simulink model "TST_DrvDem_CalcState"  (R2016b)
settings: Solver=FixedStepDiscrete  StartTime=0.0  StopTime=simTime  FixedStep=sampleTime  RelTol=1e-3
values from neighbouring files (symbols this model uses):
  testCase = 1    [initTST_DrvDem_CalcState_001.m]    (also in initTST_DrvDem_CalcState_002.m = 2)
libraries: simulink x11, UnitTest_Lib x8
settings Model: Creator=zhengjinyan  LastModifiedBy=zhengjinyan
settings DebuggingCC: SignalRangeChecking=error

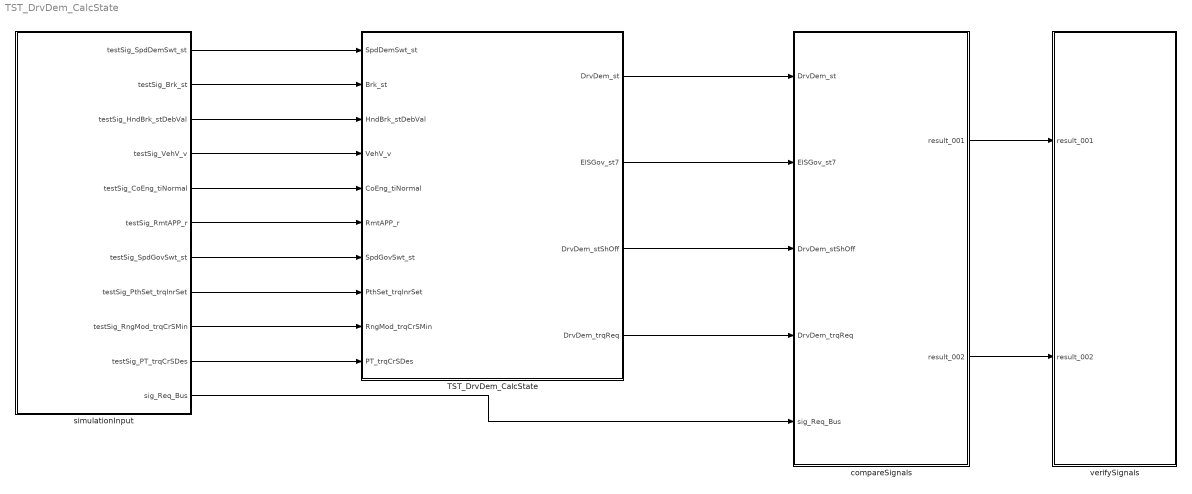
== system TST_DrvDem_CalcState ==
  TST_DrvDem_CalcState : Subsystem
  compareSignals : Subsystem
  simulationInput : Subsystem
  verifySignals : Subsystem
  wires:
  simulationInput/1(testSig_SpdDemSwt_st) -> TST_DrvDem_CalcState/1(SpdDemSwt_st)
  simulationInput/2(testSig_Brk_st) -> TST_DrvDem_CalcState/2(Brk_st)
  simulationInput/3(testSig_HndBrk_stDebVal) -> TST_DrvDem_CalcState/3(HndBrk_stDebVal)
  simulationInput/4(testSig_VehV_v) -> TST_DrvDem_CalcState/4(VehV_v)
  simulationInput/5(testSig_CoEng_tiNormal) -> TST_DrvDem_CalcState/5(CoEng_tiNormal)
  simulationInput/6(testSig_RmtAPP_r) -> TST_DrvDem_CalcState/6(RmtAPP_r)
  simulationInput/7(testSig_SpdGovSwt_st) -> TST_DrvDem_CalcState/7(SpdGovSwt_st)
  simulationInput/8(testSig_PthSet_trqInrSet) -> TST_DrvDem_CalcState/8(PthSet_trqInrSet)
  simulationInput/9(testSig_RngMod_trqCrSMin) -> TST_DrvDem_CalcState/9(RngMod_trqCrSMin)
  simulationInput/10(testSig_PT_trqCrSDes) -> TST_DrvDem_CalcState/10(PT_trqCrSDes)
  TST_DrvDem_CalcState/1(DrvDem_st) -> compareSignals/1(DrvDem_st)
  TST_DrvDem_CalcState/2(EISGov_st7) -> compareSignals/2(EISGov_st7)
  TST_DrvDem_CalcState/3(DrvDem_stShOff) -> compareSignals/3(DrvDem_stShOff)
  TST_DrvDem_CalcState/4(DrvDem_trqReq) -> compareSignals/4(DrvDem_trqReq)
  simulationInput/11(sig_Req_Bus) -> compareSignals/5(sig_Req_Bus)
  compareSignals/1(result_001) -> verifySignals/1(result_001)
  compareSignals/2(result_002) -> verifySignals/2(result_002)

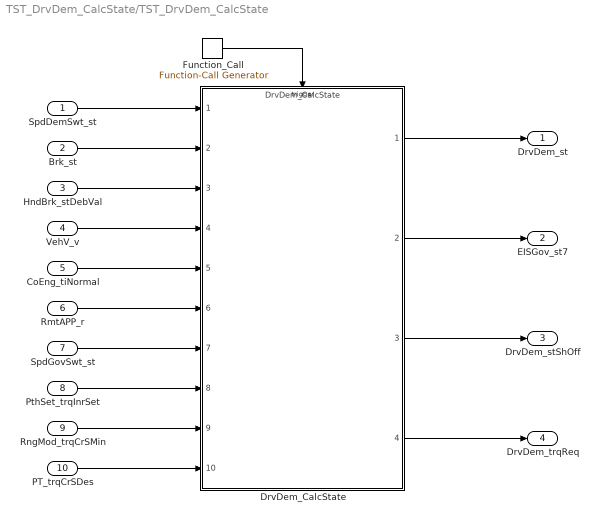
== system TST_DrvDem_CalcState/TST_DrvDem_CalcState ==
  SpdDemSwt_st : Inport
  Brk_st : Inport  Port=2
  HndBrk_stDebVal : Inport  Port=3
  VehV_v : Inport  Port=4
  CoEng_tiNormal : Inport  Port=5
  RmtAPP_r : Inport  Port=6
  SpdGovSwt_st : Inport  Port=7
  PthSet_trqInrSet : Inport  Port=8
  RngMod_trqCrSMin : Inport  Port=9
  PT_trqCrSDes : Inport  Port=10
  DrvDem_CalcState : ModelReference  ModelNameDialog=DrvDem_CalcState  SimulationMode=Normal  ModelReferenceVersion=1.66  TriggerPortName=function  TriggerPortTriggerType=function-call  TriggerPortStatesWhenEnabling=held
  Function_Call : simulink/Ports & Subsystems/Function-Call Generator  sample_time=sampleTime  numberOfIterations=1
  DrvDem_st : Outport
  EISGov_st7 : Outport  Port=2
  DrvDem_stShOff : Outport  Port=3
  DrvDem_trqReq : Outport  Port=4
  wires:
  Function_Call/1 -> DrvDem_CalcState/Trigger
  SpdDemSwt_st/1 -> DrvDem_CalcState/1
  Brk_st/1 -> DrvDem_CalcState/2
  HndBrk_stDebVal/1 -> DrvDem_CalcState/3
  VehV_v/1 -> DrvDem_CalcState/4
  CoEng_tiNormal/1 -> DrvDem_CalcState/5
  RmtAPP_r/1 -> DrvDem_CalcState/6
  SpdGovSwt_st/1 -> DrvDem_CalcState/7
  PthSet_trqInrSet/1 -> DrvDem_CalcState/8
  RngMod_trqCrSMin/1 -> DrvDem_CalcState/9
  PT_trqCrSDes/1 -> DrvDem_CalcState/10
  DrvDem_CalcState/1 -> DrvDem_st/1
  DrvDem_CalcState/2 -> EISGov_st7/1
  DrvDem_CalcState/3 -> DrvDem_stShOff/1
  DrvDem_CalcState/4 -> DrvDem_trqReq/1

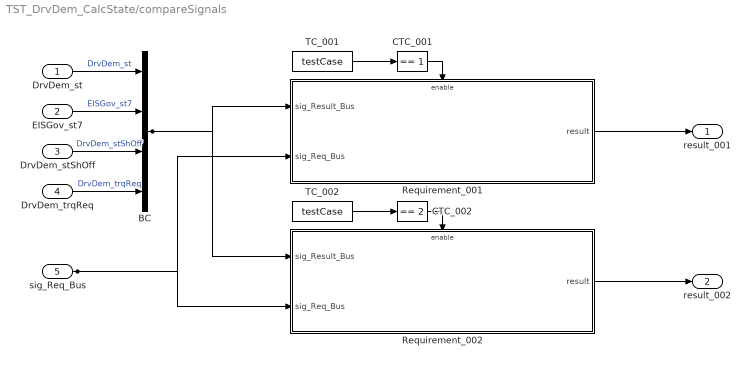
== system TST_DrvDem_CalcState/compareSignals ==
  DrvDem_st : Inport
  EISGov_st7 : Inport  Port=2
  DrvDem_stShOff : Inport  Port=3
  DrvDem_trqReq : Inport  Port=4
  sig_Req_Bus : Inport  Port=5
  BC : BusCreator  Inputs=4
  CTC_001 : simulink/Logic and Bit Operations/Compare To Constant  relop===  const=1  OutDataTypeStr=boolean
  CTC_002 : simulink/Logic and Bit Operations/Compare To Constant  relop===  const=2  OutDataTypeStr=boolean
  Requirement_001 : Subsystem
  Requirement_002 : Subsystem
  TC_001 : Constant  Value=testCase
  TC_002 : Constant  Value=testCase
  result_001 : Outport
  result_002 : Outport  Port=2
  wires:
  DrvDem_st/1 -> BC/1  "DrvDem_st"
  EISGov_st7/1 -> BC/2  "EISGov_st7"
  DrvDem_stShOff/1 -> BC/3  "DrvDem_stShOff"
  DrvDem_trqReq/1 -> BC/4  "DrvDem_trqReq"
  TC_001/1 -> CTC_001/1
  CTC_001/1 -> Requirement_001/Enable
  sig_Req_Bus/1 -> Requirement_001/2(sig_Req_Bus), Requirement_002/2(sig_Req_Bus)
  BC/1 -> Requirement_001/1(sig_Result_Bus), Requirement_002/1(sig_Result_Bus)
  Requirement_001/1(result) -> result_001/1
  TC_002/1 -> CTC_002/1
  CTC_002/1 -> Requirement_002/Enable
  Requirement_002/1(result) -> result_002/1

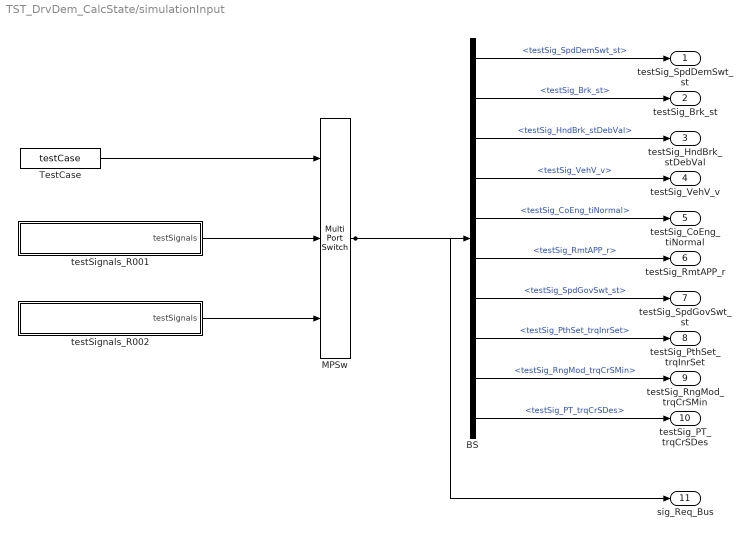
== system TST_DrvDem_CalcState/simulationInput ==
  BS : BusSelector  OutputSignals=testSig_SpdDemSwt_st,testSig_Brk_st,testSig_HndBrk_stDebVal,testSig_VehV_v,testSig_CoEng_tiNormal,testSig_RmtAPP_r,testSig_SpdGovSwt_st,testSig_PthSet_trqInrSet,testSig_RngMod_trqCrSMin,testSig_PT_trqCrSDes
  MPSw : MultiPortSwitch  Inputs=2  SaturateOnIntegerOverflow=on  InputSameDT=on
  TestCase : Constant  Value=testCase
  testSignals_R001 : Subsystem
  testSignals_R002 : Subsystem
  testSig_SpdDemSwt_st : Outport
  testSig_Brk_st : Outport  Port=2
  testSig_HndBrk_stDebVal : Outport  Port=3
  testSig_VehV_v : Outport  Port=4
  testSig_CoEng_tiNormal : Outport  Port=5
  testSig_RmtAPP_r : Outport  Port=6
  testSig_SpdGovSwt_st : Outport  Port=7
  testSig_PthSet_trqInrSet : Outport  Port=8
  testSig_RngMod_trqCrSMin : Outport  Port=9
  testSig_PT_trqCrSDes : Outport  Port=10
  sig_Req_Bus : Outport  Port=11
  wires:
  BS/1 -> testSig_SpdDemSwt_st/1  "<testSig_SpdDemSwt_st>"
  BS/2 -> testSig_Brk_st/1  "<testSig_Brk_st>"
  BS/3 -> testSig_HndBrk_stDebVal/1  "<testSig_HndBrk_stDebVal>"
  BS/4 -> testSig_VehV_v/1  "<testSig_VehV_v>"
  BS/5 -> testSig_CoEng_tiNormal/1  "<testSig_CoEng_tiNormal>"
  BS/6 -> testSig_RmtAPP_r/1  "<testSig_RmtAPP_r>"
  BS/7 -> testSig_SpdGovSwt_st/1  "<testSig_SpdGovSwt_st>"
  BS/8 -> testSig_PthSet_trqInrSet/1  "<testSig_PthSet_trqInrSet>"
  BS/9 -> testSig_RngMod_trqCrSMin/1  "<testSig_RngMod_trqCrSMin>"
  BS/10 -> testSig_PT_trqCrSDes/1  "<testSig_PT_trqCrSDes>"
  MPSw/1 -> BS/1, sig_Req_Bus/1
  TestCase/1 -> MPSw/1
  testSignals_R001/1(testSignals) -> MPSw/2
  testSignals_R002/1(testSignals) -> MPSw/3

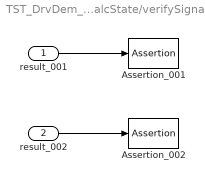
== system TST_DrvDem_CalcState/verifySignals ==
  result_001 : Inport
  result_002 : Inport  Port=2
  Assertion_001 : Assertion  Enabled=off
  Assertion_002 : Assertion  Enabled=off
  wires:
  result_001/1 -> Assertion_001/1
  result_002/1 -> Assertion_002/1

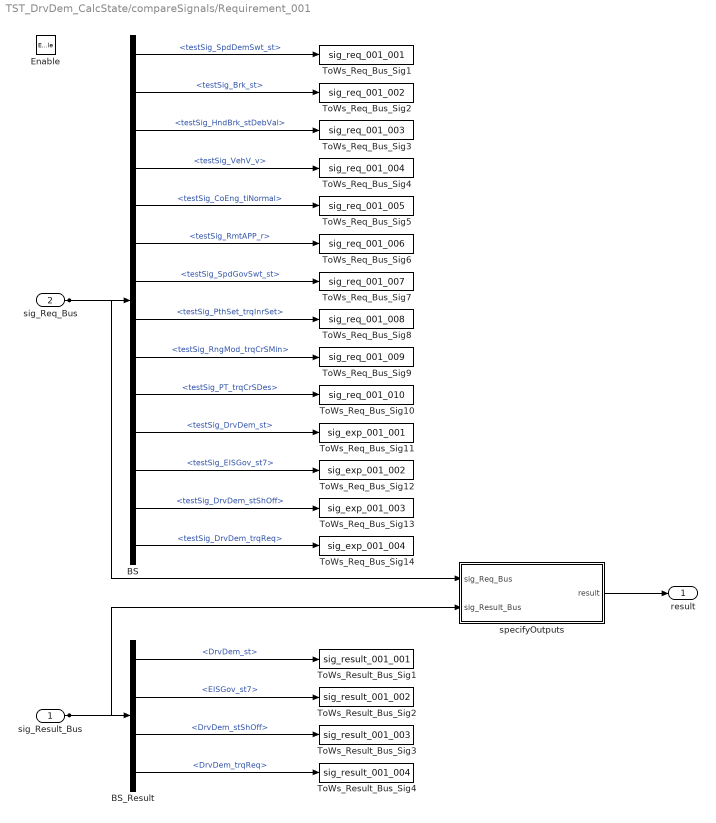
== system TST_DrvDem_CalcState/compareSignals/Requirement_001 ==
  sig_Result_Bus : Inport
  sig_Req_Bus : Inport  Port=2
  Enable : EnablePort
  BS : BusSelector  OutputSignals=testSig_SpdDemSwt_st,testSig_Brk_st,testSig_HndBrk_stDebVal,testSig_VehV_v,testSig_CoEng_tiNormal,testSig_RmtAPP_r,testSig_SpdGovSwt_st,testSig_PthSet_trqInrSet,testSig_RngMod_trqCrSMin,testSig_PT_trqCrSDes,testSig_DrvDem_st,testSig_EISGov_st7,testSig_DrvDem_stShOff,testSig_DrvDem_trqReq
  BS_Result : BusSelector  OutputSignals=DrvDem_st,EISGov_st7,DrvDem_stShOff,DrvDem_trqReq
  ToWs_Req_Bus_Sig1 : ToWorkspace  VariableName=sig_req_001_001  SaveFormat=Structure With Time
  ToWs_Req_Bus_Sig10 : ToWorkspace  VariableName=sig_req_001_010  SaveFormat=Structure With Time
  ToWs_Req_Bus_Sig11 : ToWorkspace  VariableName=sig_exp_001_001  SaveFormat=Structure With Time
  ToWs_Req_Bus_Sig12 : ToWorkspace  VariableName=sig_exp_001_002  SaveFormat=Structure With Time
  ToWs_Req_Bus_Sig13 : ToWorkspace  VariableName=sig_exp_001_003  SaveFormat=Structure With Time
  ToWs_Req_Bus_Sig14 : ToWorkspace  VariableName=sig_exp_001_004  SaveFormat=Structure With Time
  ToWs_Req_Bus_Sig2 : ToWorkspace  VariableName=sig_req_001_002  SaveFormat=Structure With Time
  ToWs_Req_Bus_Sig3 : ToWorkspace  VariableName=sig_req_001_003  SaveFormat=Structure With Time
  ToWs_Req_Bus_Sig4 : ToWorkspace  VariableName=sig_req_001_004  SaveFormat=Structure With Time
  ToWs_Req_Bus_Sig5 : ToWorkspace  VariableName=sig_req_001_005  SaveFormat=Structure With Time
  ToWs_Req_Bus_Sig6 : ToWorkspace  VariableName=sig_req_001_006  SaveFormat=Structure With Time
  ToWs_Req_Bus_Sig7 : ToWorkspace  VariableName=sig_req_001_007  SaveFormat=Structure With Time
  ToWs_Req_Bus_Sig8 : ToWorkspace  VariableName=sig_req_001_008  SaveFormat=Structure With Time
  ToWs_Req_Bus_Sig9 : ToWorkspace  VariableName=sig_req_001_009  SaveFormat=Structure With Time
  ToWs_Result_Bus_Sig1 : ToWorkspace  VariableName=sig_result_001_001  SaveFormat=Structure With Time
  ToWs_Result_Bus_Sig2 : ToWorkspace  VariableName=sig_result_001_002  SaveFormat=Structure With Time
  ToWs_Result_Bus_Sig3 : ToWorkspace  VariableName=sig_result_001_003  SaveFormat=Structure With Time
  ToWs_Result_Bus_Sig4 : ToWorkspace  VariableName=sig_result_001_004  SaveFormat=Structure With Time
  specifyOutputs : Subsystem
  result : Outport
  wires:
  sig_Req_Bus/1 -> BS/1, specifyOutputs/1(sig_Req_Bus)
  BS/1 -> ToWs_Req_Bus_Sig1/1  "<testSig_SpdDemSwt_st>"
  BS/2 -> ToWs_Req_Bus_Sig2/1  "<testSig_Brk_st>"
  BS/3 -> ToWs_Req_Bus_Sig3/1  "<testSig_HndBrk_stDebVal>"
  BS/4 -> ToWs_Req_Bus_Sig4/1  "<testSig_VehV_v>"
  BS/5 -> ToWs_Req_Bus_Sig5/1  "<testSig_CoEng_tiNormal>"
  BS/6 -> ToWs_Req_Bus_Sig6/1  "<testSig_RmtAPP_r>"
  BS/7 -> ToWs_Req_Bus_Sig7/1  "<testSig_SpdGovSwt_st>"
  BS/8 -> ToWs_Req_Bus_Sig8/1  "<testSig_PthSet_trqInrSet>"
  BS/9 -> ToWs_Req_Bus_Sig9/1  "<testSig_RngMod_trqCrSMin>"
  BS/10 -> ToWs_Req_Bus_Sig10/1  "<testSig_PT_trqCrSDes>"
  BS/11 -> ToWs_Req_Bus_Sig11/1  "<testSig_DrvDem_st>"
  BS/12 -> ToWs_Req_Bus_Sig12/1  "<testSig_EISGov_st7>"
  BS/13 -> ToWs_Req_Bus_Sig13/1  "<testSig_DrvDem_stShOff>"
  BS/14 -> ToWs_Req_Bus_Sig14/1  "<testSig_DrvDem_trqReq>"
  sig_Result_Bus/1 -> BS_Result/1, specifyOutputs/2(sig_Result_Bus)
  BS_Result/1 -> ToWs_Result_Bus_Sig1/1  "<DrvDem_st>"
  BS_Result/2 -> ToWs_Result_Bus_Sig2/1  "<EISGov_st7>"
  BS_Result/3 -> ToWs_Result_Bus_Sig3/1  "<DrvDem_stShOff>"
  BS_Result/4 -> ToWs_Result_Bus_Sig4/1  "<DrvDem_trqReq>"
  specifyOutputs/1(result) -> result/1

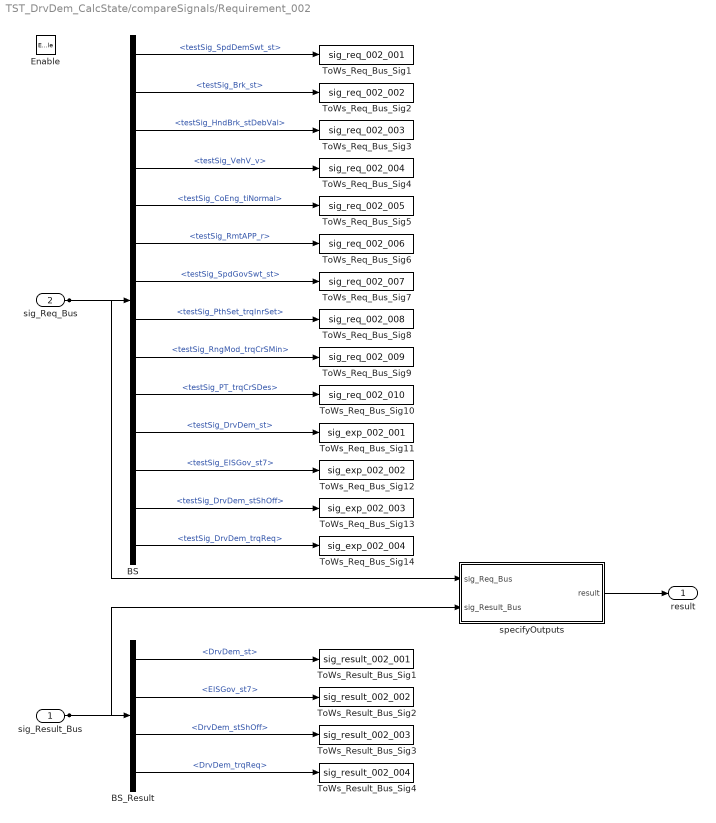
== system TST_DrvDem_CalcState/compareSignals/Requirement_002 ==
  sig_Result_Bus : Inport
  sig_Req_Bus : Inport  Port=2
  Enable : EnablePort
  BS : BusSelector  OutputSignals=testSig_SpdDemSwt_st,testSig_Brk_st,testSig_HndBrk_stDebVal,testSig_VehV_v,testSig_CoEng_tiNormal,testSig_RmtAPP_r,testSig_SpdGovSwt_st,testSig_PthSet_trqInrSet,testSig_RngMod_trqCrSMin,testSig_PT_trqCrSDes,testSig_DrvDem_st,testSig_EISGov_st7,testSig_DrvDem_stShOff,testSig_DrvDem_trqReq
  BS_Result : BusSelector  OutputSignals=DrvDem_st,EISGov_st7,DrvDem_stShOff,DrvDem_trqReq
  ToWs_Req_Bus_Sig1 : ToWorkspace  VariableName=sig_req_002_001  SaveFormat=Structure With Time
  ToWs_Req_Bus_Sig10 : ToWorkspace  VariableName=sig_req_002_010  SaveFormat=Structure With Time
  ToWs_Req_Bus_Sig11 : ToWorkspace  VariableName=sig_exp_002_001  SaveFormat=Structure With Time
  ToWs_Req_Bus_Sig12 : ToWorkspace  VariableName=sig_exp_002_002  SaveFormat=Structure With Time
  ToWs_Req_Bus_Sig13 : ToWorkspace  VariableName=sig_exp_002_003  SaveFormat=Structure With Time
  ToWs_Req_Bus_Sig14 : ToWorkspace  VariableName=sig_exp_002_004  SaveFormat=Structure With Time
  ToWs_Req_Bus_Sig2 : ToWorkspace  VariableName=sig_req_002_002  SaveFormat=Structure With Time
  ToWs_Req_Bus_Sig3 : ToWorkspace  VariableName=sig_req_002_003  SaveFormat=Structure With Time
  ToWs_Req_Bus_Sig4 : ToWorkspace  VariableName=sig_req_002_004  SaveFormat=Structure With Time
  ToWs_Req_Bus_Sig5 : ToWorkspace  VariableName=sig_req_002_005  SaveFormat=Structure With Time
  ToWs_Req_Bus_Sig6 : ToWorkspace  VariableName=sig_req_002_006  SaveFormat=Structure With Time
  ToWs_Req_Bus_Sig7 : ToWorkspace  VariableName=sig_req_002_007  SaveFormat=Structure With Time
  ToWs_Req_Bus_Sig8 : ToWorkspace  VariableName=sig_req_002_008  SaveFormat=Structure With Time
  ToWs_Req_Bus_Sig9 : ToWorkspace  VariableName=sig_req_002_009  SaveFormat=Structure With Time
  ToWs_Result_Bus_Sig1 : ToWorkspace  VariableName=sig_result_002_001  SaveFormat=Structure With Time
  ToWs_Result_Bus_Sig2 : ToWorkspace  VariableName=sig_result_002_002  SaveFormat=Structure With Time
  ToWs_Result_Bus_Sig3 : ToWorkspace  VariableName=sig_result_002_003  SaveFormat=Structure With Time
  ToWs_Result_Bus_Sig4 : ToWorkspace  VariableName=sig_result_002_004  SaveFormat=Structure With Time
  specifyOutputs : Subsystem
  result : Outport
  wires:
  sig_Req_Bus/1 -> BS/1, specifyOutputs/1(sig_Req_Bus)
  BS/1 -> ToWs_Req_Bus_Sig1/1  "<testSig_SpdDemSwt_st>"
  BS/2 -> ToWs_Req_Bus_Sig2/1  "<testSig_Brk_st>"
  BS/3 -> ToWs_Req_Bus_Sig3/1  "<testSig_HndBrk_stDebVal>"
  BS/4 -> ToWs_Req_Bus_Sig4/1  "<testSig_VehV_v>"
  BS/5 -> ToWs_Req_Bus_Sig5/1  "<testSig_CoEng_tiNormal>"
  BS/6 -> ToWs_Req_Bus_Sig6/1  "<testSig_RmtAPP_r>"
  BS/7 -> ToWs_Req_Bus_Sig7/1  "<testSig_SpdGovSwt_st>"
  BS/8 -> ToWs_Req_Bus_Sig8/1  "<testSig_PthSet_trqInrSet>"
  BS/9 -> ToWs_Req_Bus_Sig9/1  "<testSig_RngMod_trqCrSMin>"
  BS/10 -> ToWs_Req_Bus_Sig10/1  "<testSig_PT_trqCrSDes>"
  BS/11 -> ToWs_Req_Bus_Sig11/1  "<testSig_DrvDem_st>"
  BS/12 -> ToWs_Req_Bus_Sig12/1  "<testSig_EISGov_st7>"
  BS/13 -> ToWs_Req_Bus_Sig13/1  "<testSig_DrvDem_stShOff>"
  BS/14 -> ToWs_Req_Bus_Sig14/1  "<testSig_DrvDem_trqReq>"
  sig_Result_Bus/1 -> BS_Result/1, specifyOutputs/2(sig_Result_Bus)
  BS_Result/1 -> ToWs_Result_Bus_Sig1/1  "<DrvDem_st>"
  BS_Result/2 -> ToWs_Result_Bus_Sig2/1  "<EISGov_st7>"
  BS_Result/3 -> ToWs_Result_Bus_Sig3/1  "<DrvDem_stShOff>"
  BS_Result/4 -> ToWs_Result_Bus_Sig4/1  "<DrvDem_trqReq>"
  specifyOutputs/1(result) -> result/1

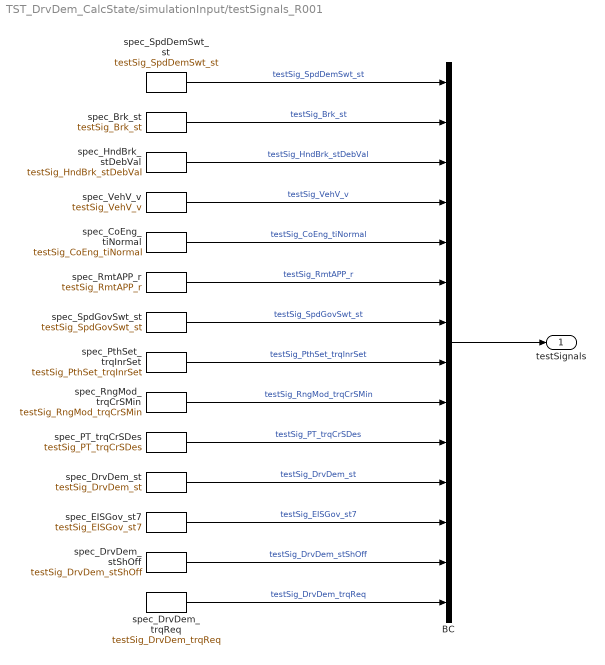
== system TST_DrvDem_CalcState/simulationInput/testSignals_R001 ==
  BC : BusCreator  Inputs=14
  spec_Brk_st : FromWorkspace  VariableName=testSig_Brk_st  Interpolate=off  OutputAfterFinalValue=Holding final value
  spec_CoEng_tiNormal : FromWorkspace  VariableName=testSig_CoEng_tiNormal  Interpolate=off  OutputAfterFinalValue=Holding final value
  spec_DrvDem_st : FromWorkspace  VariableName=testSig_DrvDem_st  Interpolate=off  OutputAfterFinalValue=Holding final value
  spec_DrvDem_stShOff : FromWorkspace  VariableName=testSig_DrvDem_stShOff  Interpolate=off  OutputAfterFinalValue=Holding final value
  spec_DrvDem_trqReq : FromWorkspace  VariableName=testSig_DrvDem_trqReq  Interpolate=off  OutputAfterFinalValue=Holding final value
  spec_EISGov_st7 : FromWorkspace  VariableName=testSig_EISGov_st7  Interpolate=off  OutputAfterFinalValue=Holding final value
  spec_HndBrk_stDebVal : FromWorkspace  VariableName=testSig_HndBrk_stDebVal  Interpolate=off  OutputAfterFinalValue=Holding final value
  spec_PT_trqCrSDes : FromWorkspace  VariableName=testSig_PT_trqCrSDes  Interpolate=off  OutputAfterFinalValue=Holding final value
  spec_PthSet_trqInrSet : FromWorkspace  VariableName=testSig_PthSet_trqInrSet  Interpolate=off  OutputAfterFinalValue=Holding final value
  spec_RmtAPP_r : FromWorkspace  VariableName=testSig_RmtAPP_r  Interpolate=off  OutputAfterFinalValue=Holding final value
  spec_RngMod_trqCrSMin : FromWorkspace  VariableName=testSig_RngMod_trqCrSMin  Interpolate=off  OutputAfterFinalValue=Holding final value
  spec_SpdDemSwt_st : FromWorkspace  VariableName=testSig_SpdDemSwt_st  Interpolate=off  OutputAfterFinalValue=Holding final value
  spec_SpdGovSwt_st : FromWorkspace  VariableName=testSig_SpdGovSwt_st  Interpolate=off  OutputAfterFinalValue=Holding final value
  spec_VehV_v : FromWorkspace  VariableName=testSig_VehV_v  Interpolate=off  OutputAfterFinalValue=Holding final value
  testSignals : Outport
  wires:
  BC/1 -> testSignals/1
  spec_SpdDemSwt_st/1 -> BC/1  "testSig_SpdDemSwt_st"
  spec_Brk_st/1 -> BC/2  "testSig_Brk_st"
  spec_HndBrk_stDebVal/1 -> BC/3  "testSig_HndBrk_stDebVal"
  spec_VehV_v/1 -> BC/4  "testSig_VehV_v"
  spec_CoEng_tiNormal/1 -> BC/5  "testSig_CoEng_tiNormal"
  spec_RmtAPP_r/1 -> BC/6  "testSig_RmtAPP_r"
  spec_SpdGovSwt_st/1 -> BC/7  "testSig_SpdGovSwt_st"
  spec_PthSet_trqInrSet/1 -> BC/8  "testSig_PthSet_trqInrSet"
  spec_RngMod_trqCrSMin/1 -> BC/9  "testSig_RngMod_trqCrSMin"
  spec_PT_trqCrSDes/1 -> BC/10  "testSig_PT_trqCrSDes"
  spec_DrvDem_st/1 -> BC/11  "testSig_DrvDem_st"
  spec_EISGov_st7/1 -> BC/12  "testSig_EISGov_st7"
  spec_DrvDem_stShOff/1 -> BC/13  "testSig_DrvDem_stShOff"
  spec_DrvDem_trqReq/1 -> BC/14  "testSig_DrvDem_trqReq"

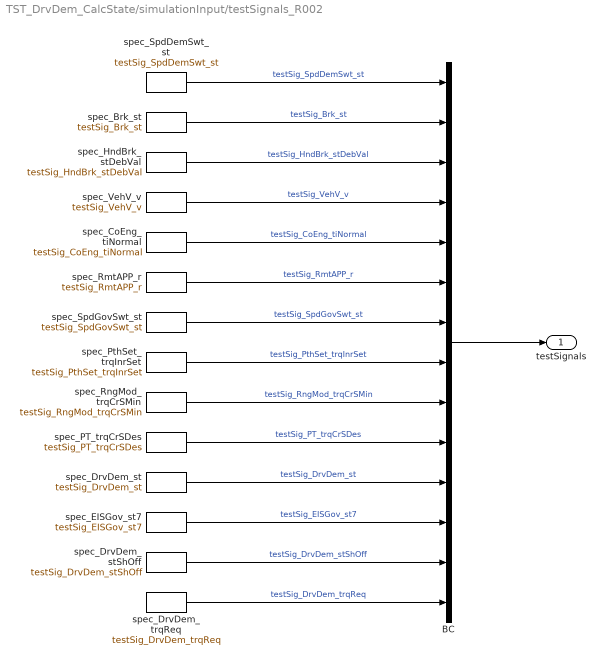
== system TST_DrvDem_CalcState/simulationInput/testSignals_R002 ==
  BC : BusCreator  Inputs=14
  spec_Brk_st : FromWorkspace  VariableName=testSig_Brk_st  Interpolate=off  OutputAfterFinalValue=Holding final value
  spec_CoEng_tiNormal : FromWorkspace  VariableName=testSig_CoEng_tiNormal  Interpolate=off  OutputAfterFinalValue=Holding final value
  spec_DrvDem_st : FromWorkspace  VariableName=testSig_DrvDem_st  Interpolate=off  OutputAfterFinalValue=Holding final value
  spec_DrvDem_stShOff : FromWorkspace  VariableName=testSig_DrvDem_stShOff  Interpolate=off  OutputAfterFinalValue=Holding final value
  spec_DrvDem_trqReq : FromWorkspace  VariableName=testSig_DrvDem_trqReq  Interpolate=off  OutputAfterFinalValue=Holding final value
  spec_EISGov_st7 : FromWorkspace  VariableName=testSig_EISGov_st7  Interpolate=off  OutputAfterFinalValue=Holding final value
  spec_HndBrk_stDebVal : FromWorkspace  VariableName=testSig_HndBrk_stDebVal  Interpolate=off  OutputAfterFinalValue=Holding final value
  spec_PT_trqCrSDes : FromWorkspace  VariableName=testSig_PT_trqCrSDes  Interpolate=off  OutputAfterFinalValue=Holding final value
  spec_PthSet_trqInrSet : FromWorkspace  VariableName=testSig_PthSet_trqInrSet  Interpolate=off  OutputAfterFinalValue=Holding final value
  spec_RmtAPP_r : FromWorkspace  VariableName=testSig_RmtAPP_r  Interpolate=off  OutputAfterFinalValue=Holding final value
  spec_RngMod_trqCrSMin : FromWorkspace  VariableName=testSig_RngMod_trqCrSMin  Interpolate=off  OutputAfterFinalValue=Holding final value
  spec_SpdDemSwt_st : FromWorkspace  VariableName=testSig_SpdDemSwt_st  Interpolate=off  OutputAfterFinalValue=Holding final value
  spec_SpdGovSwt_st : FromWorkspace  VariableName=testSig_SpdGovSwt_st  Interpolate=off  OutputAfterFinalValue=Holding final value
  spec_VehV_v : FromWorkspace  VariableName=testSig_VehV_v  Interpolate=off  OutputAfterFinalValue=Holding final value
  testSignals : Outport
  wires:
  BC/1 -> testSignals/1
  spec_SpdDemSwt_st/1 -> BC/1  "testSig_SpdDemSwt_st"
  spec_Brk_st/1 -> BC/2  "testSig_Brk_st"
  spec_HndBrk_stDebVal/1 -> BC/3  "testSig_HndBrk_stDebVal"
  spec_VehV_v/1 -> BC/4  "testSig_VehV_v"
  spec_CoEng_tiNormal/1 -> BC/5  "testSig_CoEng_tiNormal"
  spec_RmtAPP_r/1 -> BC/6  "testSig_RmtAPP_r"
  spec_SpdGovSwt_st/1 -> BC/7  "testSig_SpdGovSwt_st"
  spec_PthSet_trqInrSet/1 -> BC/8  "testSig_PthSet_trqInrSet"
  spec_RngMod_trqCrSMin/1 -> BC/9  "testSig_RngMod_trqCrSMin"
  spec_PT_trqCrSDes/1 -> BC/10  "testSig_PT_trqCrSDes"
  spec_DrvDem_st/1 -> BC/11  "testSig_DrvDem_st"
  spec_EISGov_st7/1 -> BC/12  "testSig_EISGov_st7"
  spec_DrvDem_stShOff/1 -> BC/13  "testSig_DrvDem_stShOff"
  spec_DrvDem_trqReq/1 -> BC/14  "testSig_DrvDem_trqReq"

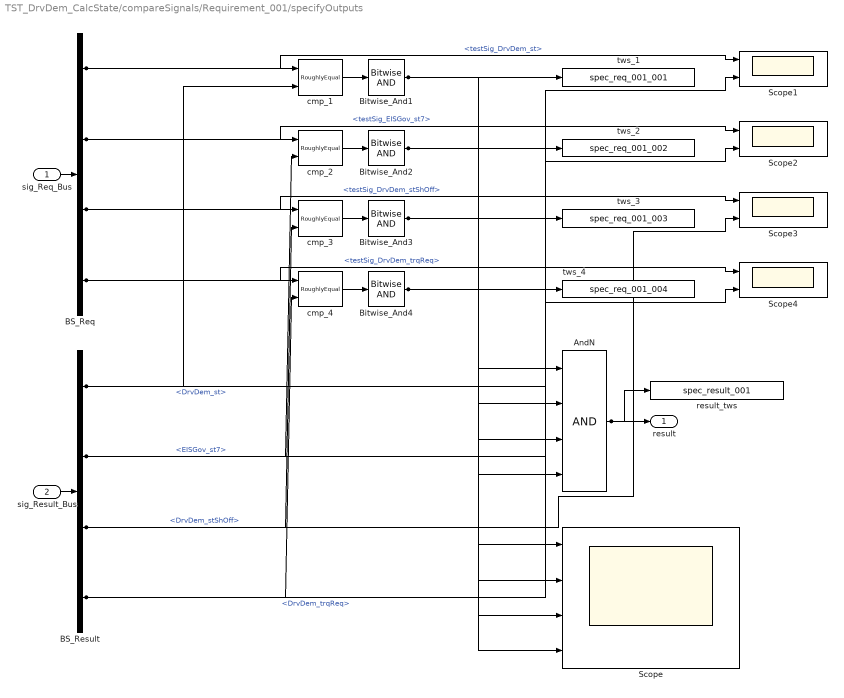
== system TST_DrvDem_CalcState/compareSignals/Requirement_001/specifyOutputs ==
  sig_Req_Bus : Inport
  sig_Result_Bus : Inport  Port=2
  AndN : Logic  Inputs=4
  BS_Req : BusSelector  OutputSignals=testSig_DrvDem_st,testSig_EISGov_st7,testSig_DrvDem_stShOff,testSig_DrvDem_trqReq
  BS_Result : BusSelector  OutputSignals=DrvDem_st,EISGov_st7,DrvDem_stShOff,DrvDem_trqReq
  Bitwise_And{1..4} (4 alike) : simulink/Logic and Bit Operations/Bitwise Operator  logicop=AND  UseBitMask=off  BitMask=bin2dec('11011001')  BitMaskRealWorld=Stored Integer
  Scope : Scope  NumInputPorts=4
  Scope{1..4} (4 alike) : Scope  NumInputPorts=2
  cmp_{1..4} (4 alike) : UnitTest_Lib/RoughlyEqual  slope=0.1
  result_tws : ToWorkspace  VariableName=spec_result_001
  tws_1 : ToWorkspace  VariableName=spec_req_001_001
  tws_2 : ToWorkspace  VariableName=spec_req_001_002
  tws_3 : ToWorkspace  VariableName=spec_req_001_003
  tws_4 : ToWorkspace  VariableName=spec_req_001_004
  result : Outport
  wires:
  sig_Req_Bus/1 -> BS_Req/1
  sig_Result_Bus/1 -> BS_Result/1
  AndN/1 -> result/1, result_tws/1
  BS_Req/1 -> cmp_1/1, Scope1/1  "<testSig_DrvDem_st>"
  BS_Result/1 -> cmp_1/2, Scope1/2  "<DrvDem_st>"
  cmp_1/1 -> Bitwise_And1/1
  Bitwise_And1/1 -> tws_1/1, AndN/1, Scope/1
  BS_Req/2 -> cmp_2/1, Scope2/1  "<testSig_EISGov_st7>"
  BS_Result/2 -> cmp_2/2, Scope2/2  "<EISGov_st7>"
  cmp_2/1 -> Bitwise_And2/1
  Bitwise_And2/1 -> tws_2/1, AndN/2, Scope/2
  BS_Req/3 -> cmp_3/1, Scope3/1  "<testSig_DrvDem_stShOff>"
  BS_Result/3 -> cmp_3/2, Scope3/2  "<DrvDem_stShOff>"
  cmp_3/1 -> Bitwise_And3/1
  Bitwise_And3/1 -> tws_3/1, AndN/3, Scope/3
  BS_Req/4 -> cmp_4/1, Scope4/1  "<testSig_DrvDem_trqReq>"
  BS_Result/4 -> cmp_4/2, Scope4/2  "<DrvDem_trqReq>"
  cmp_4/1 -> Bitwise_And4/1
  Bitwise_And4/1 -> tws_4/1, AndN/4, Scope/4

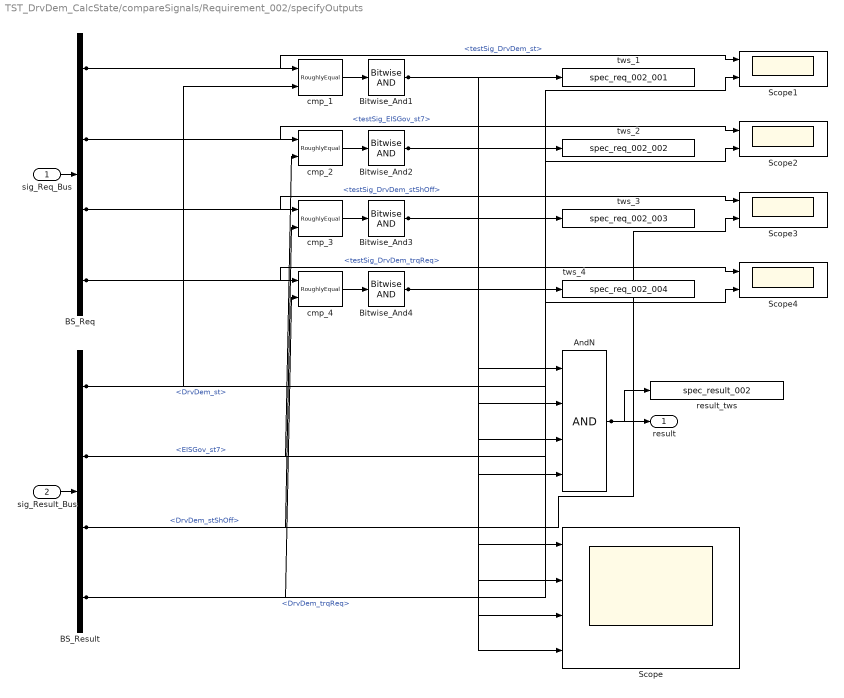
== system TST_DrvDem_CalcState/compareSignals/Requirement_002/specifyOutputs ==
  sig_Req_Bus : Inport
  sig_Result_Bus : Inport  Port=2
  AndN : Logic  Inputs=4
  BS_Req : BusSelector  OutputSignals=testSig_DrvDem_st,testSig_EISGov_st7,testSig_DrvDem_stShOff,testSig_DrvDem_trqReq
  BS_Result : BusSelector  OutputSignals=DrvDem_st,EISGov_st7,DrvDem_stShOff,DrvDem_trqReq
  Bitwise_And{1..4} (4 alike) : simulink/Logic and Bit Operations/Bitwise Operator  logicop=AND  UseBitMask=off  BitMask=bin2dec('11011001')  BitMaskRealWorld=Stored Integer
  Scope : Scope  NumInputPorts=4
  Scope{1..4} (4 alike) : Scope  NumInputPorts=2
  cmp_{1..4} (4 alike) : UnitTest_Lib/RoughlyEqual  slope=0.1
  result_tws : ToWorkspace  VariableName=spec_result_002
  tws_1 : ToWorkspace  VariableName=spec_req_002_001
  tws_2 : ToWorkspace  VariableName=spec_req_002_002
  tws_3 : ToWorkspace  VariableName=spec_req_002_003
  tws_4 : ToWorkspace  VariableName=spec_req_002_004
  result : Outport
  wires:
  sig_Req_Bus/1 -> BS_Req/1
  sig_Result_Bus/1 -> BS_Result/1
  AndN/1 -> result/1, result_tws/1
  BS_Req/1 -> cmp_1/1, Scope1/1  "<testSig_DrvDem_st>"
  BS_Result/1 -> cmp_1/2, Scope1/2  "<DrvDem_st>"
  cmp_1/1 -> Bitwise_And1/1
  Bitwise_And1/1 -> tws_1/1, AndN/1, Scope/1
  BS_Req/2 -> cmp_2/1, Scope2/1  "<testSig_EISGov_st7>"
  BS_Result/2 -> cmp_2/2, Scope2/2  "<EISGov_st7>"
  cmp_2/1 -> Bitwise_And2/1
  Bitwise_And2/1 -> tws_2/1, AndN/2, Scope/2
  BS_Req/3 -> cmp_3/1, Scope3/1  "<testSig_DrvDem_stShOff>"
  BS_Result/3 -> cmp_3/2, Scope3/2  "<DrvDem_stShOff>"
  cmp_3/1 -> Bitwise_And3/1
  Bitwise_And3/1 -> tws_3/1, AndN/3, Scope/3
  BS_Req/4 -> cmp_4/1, Scope4/1  "<testSig_DrvDem_trqReq>"
  BS_Result/4 -> cmp_4/2, Scope4/2  "<DrvDem_trqReq>"
  cmp_4/1 -> Bitwise_And4/1
  Bitwise_And4/1 -> tws_4/1, AndN/4, Scope/4
